simulink model "Fault_ckt"  (R2022b)
settings: Solver=ode23t  StartTime=0.0  StopTime=tFinal  MaxStep=tStepMax  RelTol=1e-3
model workspace (MAT data in the model file):
  r_pul = [0.01273 0.3864]
values from neighbouring files (symbols this model uses):
  time_of_fault = 0.25    [automation_script.m]    (also in test_script.m = 0.3)
undefined symbols (not defined in the file or in its folder): D1, Delta
libraries: spsDistributedParametersLineLib x2, spsFirstOrderFilterLib x2, spsThreePhaseParallelRLCLoadLib x1, spsThreePhaseTransformerTwoWindingsLib x1, spsThreePhaseVIMeasurementLib x1, spsThreePhaseFaultLib x1, spsThreePhaseSourceLib x1, spspowerguiLib x1
settings Model: Creator=Priyanshu Ratan  LastModifiedBy=Priyanshu Ratan

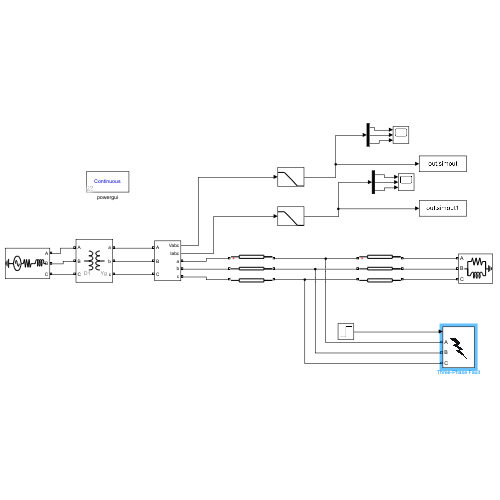
[thumbnail: Simulink's stored preview of the top-level diagram]
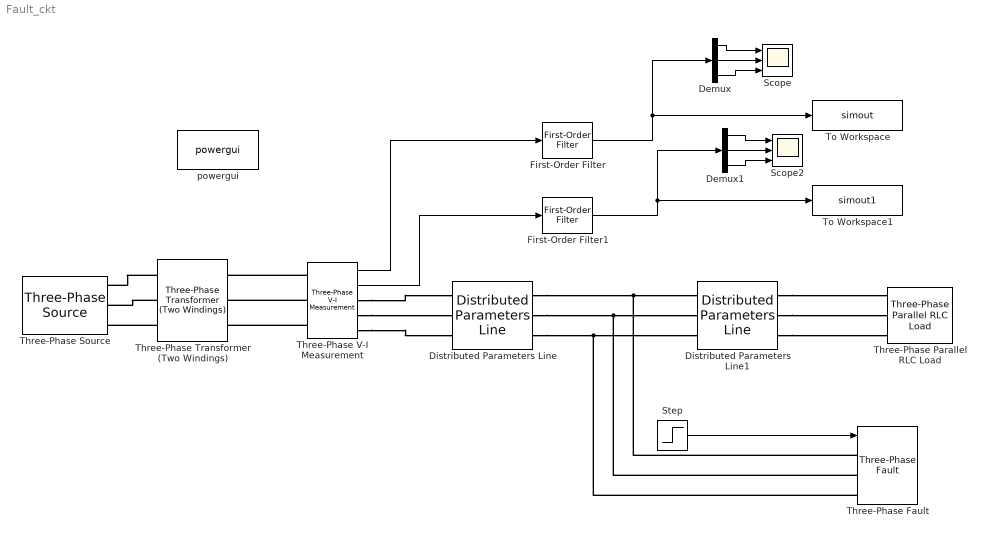
== system Fault_ckt ==
  Demux : Demux  Outputs=3
  Demux1 : Demux  Outputs=3
  Distributed Parameters Line : spsDistributedParametersLineLib/Distributed Parameters Line  Phases=3  Length=lineLength1  Frequency=50  Resistance=[0.01273 0.3864]  Inductance="[0.9337e-3  4.1264e-3]"  Capacitance=[12.74e-9 7.751e-9]  x1=[2.32281191275277e-12 399.298161194135 399.298161194132;314.159265358979 314.159265358979 314.159265358979;-2.16039013895041 1.02454669808876 -0.546249628706148]  x2=[1.92056954444993e-12 299.644393904932 299.644393904931;314.159265358979 314.159265358979 314.159265358979;-1.78486022526658 1.02406580071894 -0.546730526075966]  x3=[3.91236241558099e-14 16.9460429681368 16.9460429681366;314.159265358979 314.159265358979 314.159265358979;-1.16288201501863 2.55319884109871 0.982402514303801]  x4=[2.6870215388793e-14 17.061837324977 17.0618373249768;314.159265358979 314.159265358979 314.159265358979;2.01361473353008 -0.436663096306638 -2.00745942310154]  x5=0.000113108313399149  V1=[2.323e-12 399.3 399.3;314.2 314.2 314.2;-2.16 1.025 -0.5462]  V2=[1.921e-12 299.6 299.6;314.2 314.2 314.2;-1.785 1.024 -0.5467]  I1=[3.912e-14 16.95 16.95;314.2 314.2 314.2;-1.163 2.553 0.9824]  I2=[2.687e-14 17.06 17.06;314.2 314.2 314.2;2.014 -0.4367 -2.007]  nHarmo=1  Measurements=None  Decoupling=off  VsMag0=0  VrMag0=0  VsAngle0=0  VrAngle0=0  IsMag0=0  IrMag0=0  IsAngle0=0  IrAngle0=0
      settings: LibrarySourceBlock=sps_lib/Power Grid Elements/Distributed Parameters Line
  Distributed Parameters Line1 : spsDistributedParametersLineLib/Distributed Parameters Line  Phases=3  Length=lineLength2  Frequency=50  Resistance=[0.01273 0.3864]  Inductance="[0.9337e-3  4.1264e-3]"  Capacitance=[12.74e-9 7.751e-9]  x1=[1.92056954444993e-12 299.644393904932 299.644393904931;314.159265358979 314.159265358979 314.159265358979;-1.85592827455352 0.980724867590589 -0.590071459204314]  x2=[7.62142028251421e-16 0.544632520094194 0.544632520094191;314.159265358979 314.159265358979 314.159265358979;2.8518797623969 -0.540927046059281 -2.11172337285418]  x3=[2.44770070388107e-14 16.9460093703193 16.9460093703192;314.159265358979 314.159265358979 314.159265358979;-0.106602073930409 2.53160779186791 0.960811465073008]  x4=[2.45393689412548e-14 16.9979171080436 16.9979171080435;314.159265358979 314.159265358979 314.159265358979;3.10629804444467 -0.544926552308039 -2.11572287910294]  x5=0.000339324940197446  V1=[1.921e-12 299.6 299.6;314.2 314.2 314.2;-1.856 0.9807 -0.5901]  V2=[7.621e-16 0.5446 0.5446;314.2 314.2 314.2;2.852 -0.5409 -2.112]  I1=[2.448e-14 16.95 16.95;314.2 314.2 314.2;-0.1066 2.532 0.9608]  I2=[2.454e-14 17 17;314.2 314.2 314.2;3.106 -0.5449 -2.116]  nHarmo=1  Measurements=None  Decoupling=off  VsMag0=0  VrMag0=0  VsAngle0=0  VrAngle0=0  IsMag0=0  IrMag0=0  IsAngle0=0  IrAngle0=0
      settings: LibrarySourceBlock=sps_lib/Power Grid Elements/Distributed Parameters Line
  First-Order Filter : spsFirstOrderFilterLib/First-Order Filter  FilterType=Lowpass  Tc=10e-3  Ts=0  Initialize=on  Vac_Init=[0, 0, 60]  Vdc_Init=0  PlotResponse=off  FreqRange="[0,  200,  1]"
  First-Order Filter1 : spsFirstOrderFilterLib/First-Order Filter  FilterType=Lowpass  Tc=10e-3  Ts=0  Initialize=on  Vac_Init=[0, 0, 60]  Vdc_Init=0  PlotResponse=off  FreqRange="[0,  200,  1]"
  Scope : Scope  NumInputPorts=3
  Scope2 : Scope  NumInputPorts=3
  Step : Step  Time=time_of_fault  SampleTime=0
  Three-Phase Parallel RLC Load : spsThreePhaseParallelRLCLoadLib/Three-Phase Parallel RLC Load  LConnTagsString=A|B|C  Configuration=Y (grounded)  NominalVoltage=0.4e3  Vabc=[1e3 1e3 1e3]  Vabcp=[1e3 1e3 1e3]  NominalFrequency=50  UnbalancedPower=off  ActivePower=5e6  InductivePower=20e3  CapacitivePower=0  Pabc=[10e3 9e3 11e3]  QLabc=[100 90 110]  QCabc=[100 90 110]  Pabcp=[10e3 9e3 11e3]  QLabcp=[100 90 110]  QCabcp=[100 90 110]  Measurements=None  LoadType=constant Z
  Three-Phase Transformer (Two Windings) : spsThreePhaseTransformerTwoWindingsLib/Three-Phase Transformer (Two Windings)  Winding1Connection=Delta (D1)  Winding2Connection=Yg  CoreType=Three single-phase transformers  SetSaturation=off  Hysteresis=off  DataFile='hysteresis'  SetInitialFlux=off  Measurements=None  UNITS=pu  NominalPower=[ 10e6 , 50 ]  Winding1=[ 11e3 , 0.002 , 0.08 ]  Winding2=[ 0.4e3 , 0.002 , 0.08 ]  Rm=500  Lm=500  L0=0.5  Saturation=[ 0,0 ; 0.0024,1.2 ; 1.0,1.52 ]  InitialFluxes=[ 0.8 , -0.8 , 0.7 ]  BreakLoop=off  DiscreteSolver=Trapezoidal iterative  DataType=off  TransfoNumber=1
  Three-Phase V-I Measurement : spsThreePhaseVIMeasurementLib/Three-Phase V-I Measurement  VoltageMeasurement=phase-to-ground  SetLabelV=off  LabelV=Vabc  Vpu=off  VpuLL=off  CurrentMeasurement=yes  SetLabelI=off  LabelI=Iabc  Ipu=off  Pbase=100e6  Vbase=500e3  OutputType=Complex  PhasorSimulation=off  PSBequivalent=0
  Three-Phase Fault : spsThreePhaseFaultLib/Three-Phase Fault  InitialStates=0  FaultA=on  FaultB=on  FaultC=off  GroundFault=off  SwitchTimes="[1/60  5/60]"  External=on  SwitchStatus=NaN  FaultResistance=0.001  GroundResistance=0.01  SnubberResistance=1e6  SnubberCapacitance=inf  Measurements=None
  Three-Phase Source : spsThreePhaseSourceLib/Three-Phase Source  InternalConnection=Yg  VoltagePhases=off  Voltage=11e3  PhaseAngle=0  Voltage_phases=[25e3 25e3 25e3]/sqrt(3)  PhaseAngles_phases=[0 -120 +120]  Frequency=50  NonIdealSource=on  SpecifyImpedance=on  Resistance=0.8929  Inductance=16.58e-3  ShortCircuitLevel=20e6  BaseVoltage=11e3  XRratio=7  BusType=swing  Pref=10e3  Qref=0  Prefabc=[10e3, 10e3, 10e3]  Qrefabc=[0, 0, 0]  Qmin=-inf  Qmax=inf
  To Workspace : ToWorkspace  VariableName=simout  SaveFormat=Timeseries  SampleTime=-1
  To Workspace1 : ToWorkspace  VariableName=simout1  SaveFormat=Timeseries  SampleTime=-1
  powergui : spspowerguiLib/powergui  Priority=1  SimulationMode=Continuous  SampleTime=50e-6  frequency=60  Iterations=50  frequencyindice=50  Pbase=100e6  ErrMax=1e-4  UnitsV=kV  UnitsW=MW  buscounter=0  FunctionMessages=off  echomessages=off  EnableUseOfTLC=off  CurrentSourceSwitches=off  DisableSnubberDevices=off  DisableRonSwitches=off  DisableVfSwitches=off  DisplayEquations=off  AutomaticDiscreteSolvers=off  SolverType=Tustin/Backward Euler (TBE)  Interpol=off  ExternalGateDelay=off  methode=off  Ts=100  x0status=blocks  SPID=on  SwTol=0  HookPort=off  NonlinearTolerance=1e-4  nMaxIteration=100  ContinueOnMaxIteration=off  RestoreLinks=warning  ResistiveCurrentMeasurement=off  Frange=[0:2:500]  Ylog=off  Xlog=on  ShowGrid=off  save=off  variable=ZData  structure=0  ZoomFFT=off  StartTime=0.0  cycles=1  DisplayStyle=1  fundamental=60  FreqAxis=off  MaxFrequency=1000  frequencyindicesteady=1  RmsSteady=1  display=off
  wires:
  Demux/1 -> Scope/1
  Demux1/2 -> Scope2/2
  Demux/2 -> Scope/2
  Demux1/1 -> Scope2/1
  Step/1 -> Three-Phase Fault/1
  Demux1/3 -> Scope2/3
  Demux/3 -> Scope/3
  First-Order Filter/1 -> To Workspace/1, Demux/1
  Three-Phase V-I Measurement/1 -> First-Order Filter/1
  Three-Phase V-I Measurement/2 -> First-Order Filter1/1
  First-Order Filter1/1 -> To Workspace1/1, Demux1/1
  connections:
  Distributed Parameters Line1/RConn1 -- Three-Phase Parallel RLC Load/LConn1
  Distributed Parameters Line1/RConn2 -- Three-Phase Parallel RLC Load/LConn2
  Distributed Parameters Line1/RConn3 -- Three-Phase Parallel RLC Load/LConn3
  Three-Phase Fault/LConn2 -- Distributed Parameters Line1/LConn2 -- Distributed Parameters Line/RConn2
  Three-Phase Fault/LConn1 -- Distributed Parameters Line1/LConn1 -- Distributed Parameters Line/RConn1
  Three-Phase Fault/LConn3 -- Distributed Parameters Line/RConn3 -- Distributed Parameters Line1/LConn3
  Three-Phase Transformer (Two Windings)/LConn1 -- Three-Phase Source/RConn1
  Three-Phase Transformer (Two Windings)/LConn2 -- Three-Phase Source/RConn2
  Three-Phase Transformer (Two Windings)/LConn3 -- Three-Phase Source/RConn3
  Three-Phase V-I Measurement/LConn2 -- Three-Phase Transformer (Two Windings)/RConn2
  Three-Phase V-I Measurement/LConn1 -- Three-Phase Transformer (Two Windings)/RConn1
  Three-Phase V-I Measurement/LConn3 -- Three-Phase Transformer (Two Windings)/RConn3
  Three-Phase V-I Measurement/RConn1 -- Distributed Parameters Line/LConn1
  Three-Phase V-I Measurement/RConn2 -- Distributed Parameters Line/LConn2
  Three-Phase V-I Measurement/RConn3 -- Distributed Parameters Line/LConn3
